simulink model "BehSupervisor"  (R2026a)
settings: Solver=VariableStepAuto
model workspace (MAT data in the model file):
  NumLines = 4
undefined symbols (not defined in the file): PLANT_DEGRADED, PLANT_HALTED, PLANT_RUNNING, PLANT_STARTUP
settings Model: DataDictionary=BehParamsCommon.sldd  ParameterArgumentNames=NumLines  Creator=sarah  LastModifiedBy=sarah

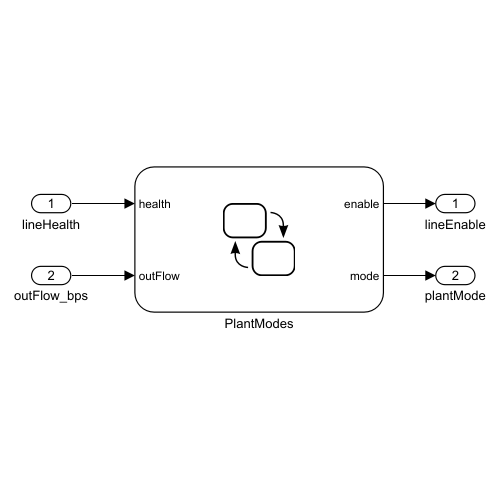
[thumbnail: Simulink's stored preview of the top-level diagram]
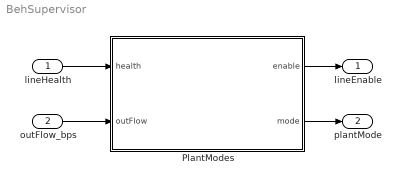
== system BehSupervisor ==
  lineHealth : Inport  PortDimensions=4
  outFlow_bps : Inport  Port=2
  PlantModes : Stateflow chart  TreatAsAtomicUnit=on
  lineEnable : Outport  PortDimensions=4
  plantMode : Outport  Port=2
  wires:
  PlantModes/2(mode) -> plantMode/1
  lineHealth/1 -> PlantModes/1(health)
  outFlow_bps/1 -> PlantModes/2(outFlow)
  PlantModes/1(enable) -> lineEnable/1

== stateflow chart BehSupervisor/PlantModes ==
  settings: updateMethod=DISCRETE  sampleTime=1
  state Startup
    du: enable = ones(1,4); mode = PLANT_STARTUP;
  state Running
    du: enable = double(health > 0.5); mode = PLANT_RUNNING;
  state Degraded
    du: enable = double(health > 0.5); mode = PLANT_DEGRADED;
  state Halted
    du: enable = zeros(1,4); mode = PLANT_HALTED;
  (default) -> Startup
  Startup -> Running : [outFlow > 0.001]
  Degraded -> Running [order 2] : [sum(health(1:NumLines) > 0.5) == NumLines]
  Running -> Degraded : [sum(health(1:NumLines) > 0.5) < NumLines]
  Halted -> Degraded : [sum(health(1:NumLines) > 0.5) > 0]
  Degraded -> Halted [order 1] : [sum(health(1:NumLines) > 0.5) == 0]
  data: health input double size=[1 4]; outFlow input double; enable output double size=[1 4]; mode output uint8; NumLines parameter double; PLANT_STARTUP parameter uint8; PLANT_RUNNING parameter uint8; PLANT_DEGRADED parameter uint8; PLANT_HALTED parameter uint8
